simulink subsystem "control_moments"  (R2021b)
settings: Solver=VariableStepAuto  StartTime=0.0  StopTime=10.0  RelTol=1e-3
libraries: vrlib x4
settings Model: Creator=austm  LastModifiedBy=austm

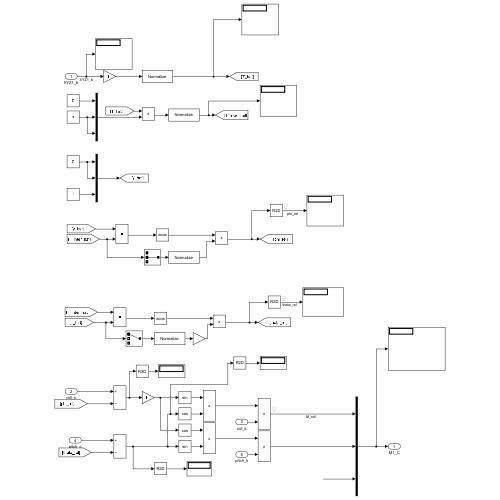
[thumbnail: Simulink's stored preview of the top-level diagram]
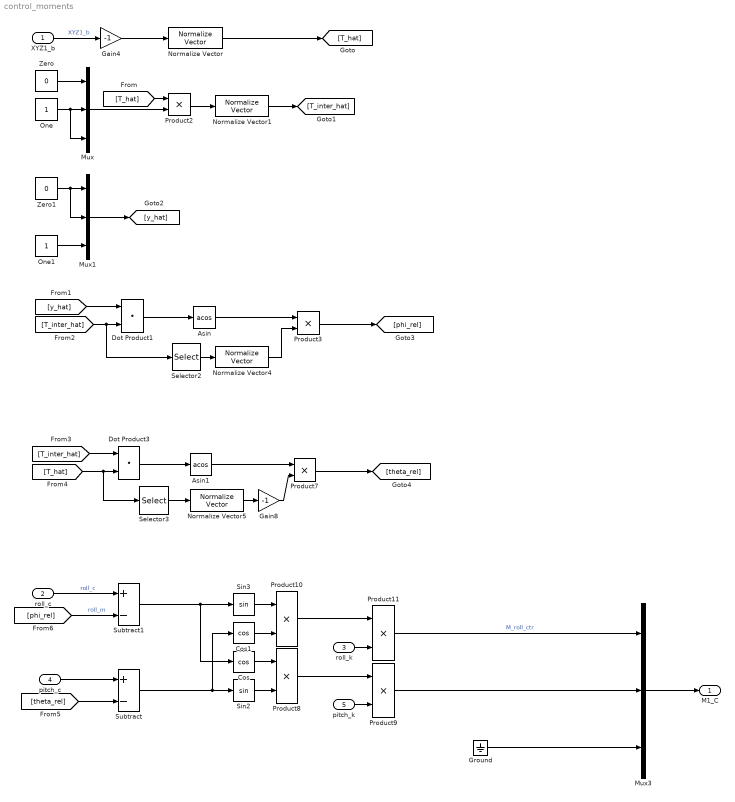
== system control_moments ==
  XYZ1_b : Inport
  roll_c : Inport  Port=2
  roll_k : Inport  Port=3
  pitch_c : Inport  Port=4
  pitch_k : Inport  Port=5
  Asin : Trigonometry  Operator=acos
  Asin1 : Trigonometry  Operator=acos
  Cos : Trigonometry  Operator=cos
  Cos1 : Trigonometry  Operator=cos
  Dot Product1 : DotProduct  InputSameDT=on  OutDataTypeStr=Inherit: Inherit via internal rule
  Dot Product3 : DotProduct  InputSameDT=on  OutDataTypeStr=Inherit: Inherit via internal rule
  Gain4 : Gain  Gain=-1
  Gain8 : Gain  Gain=-1
  Ground : Ground
  Mux : Mux  Inputs=3
  Mux1 : Mux  Inputs=3
  Mux3 : Mux  Inputs=3
  Normalize Vector{,1,4..5} (4 alike) : vrlib/Utilities/Normalize Vector  maxzero=0
  One : Constant  OutDataTypeStr=Inherit: Inherit via back propagation
  One1 : Constant  OutDataTypeStr=Inherit: Inherit via back propagation
  Product{2..3,7..11} (7 alike) : Product
  Selector2 : Selector  InputPortWidth=3  IndexOptions=Index vector (dialog)  Indices=[2]  OutputSizes=1
  Selector3 : Selector  InputPortWidth=3  IndexOptions=Index vector (dialog)  Indices=[1]  OutputSizes=1
  Sin2 : Trigonometry
  Sin3 : Trigonometry
  Subtract : Sum  Inputs=+-
  Subtract1 : Sum  Inputs=+-
  Zero : Constant  Value=0  OutDataTypeStr=Inherit: Inherit via back propagation
  Zero1 : Constant  Value=0  OutDataTypeStr=Inherit: Inherit via back propagation
  M1_C : Outport
  wires:
  Gain8/1 -> Product7/2
  Ground/1 -> Mux3/3
  Subtract1/1 -> Cos/1, Sin3/1
  Subtract/1 -> Sin2/1, Cos1/1
  Product9/1 -> Mux3/2
  Product11/1 -> Mux3/1  "M_roll_ctr"
  Mux3/1 -> M1_C/1
  roll_k/1 -> Product11/2
  Sin3/1 -> Product10/1
  Product10/1 -> Product11/1
  Cos1/1 -> Product10/2
  Product8/1 -> Product9/1
  pitch_k/1 -> Product9/2
  Cos/1 -> Product8/1
  Sin2/1 -> Product8/2
  roll_c/1 -> Subtract1/1  "roll_c"
  [phi_rel] -> Subtract1/2  "roll_m"
  pitch_c/1 -> Subtract/1
  [theta_rel] -> Subtract/2
  Asin1/1 -> Product7/1
  Normalize Vector/1 -> [T_hat]
  Selector3/1 -> Normalize Vector5/1
  Normalize Vector5/1 -> Gain8/1
  Normalize Vector4/1 -> Product3/2
  Asin/1 -> Product3/1
  Selector2/1 -> Normalize Vector4/1
  Normalize Vector1/1 -> [T_inter_hat]
  Dot Product3/1 -> Asin1/1
  [T_inter_hat] -> Dot Product3/1
  Product7/1 -> [theta_rel]
  [T_hat] -> Selector3/1, Dot Product3/2
  Product3/1 -> [phi_rel]
  [T_inter_hat] -> Selector2/1, Dot Product1/2
  [y_hat] -> Dot Product1/1
  Dot Product1/1 -> Asin/1
  Mux1/1 -> [y_hat]
  One1/1 -> Mux1/3
  Zero1/1 -> Mux1/2, Mux1/1
  Product2/1 -> Normalize Vector1/1
  [T_hat] -> Product2/1
  Mux/1 -> Product2/2
  One/1 -> Mux/3, Mux/2
  Zero/1 -> Mux/1
  Gain4/1 -> Normalize Vector/1
  XYZ1_b/1 -> Gain4/1  "XYZ1_b"
